simulink model "pndo_org"  (Simulink 10.0)
settings: Solver=ode23tb  StartTime=0.0  StopTime=12  RelTol=1e-3  EnableMultiTasking=on
undefined symbols (not defined in the file): Ts_Control
libraries: powerlib x6, re_lib x1
settings Model: Creator=Student  LastModifiedBy=annonymous
settings DataIOCC: LimitDataPoints=on  SignalLoggingSaveFormat=ModelDataLogs
settings OptimizationCC: ExpressionDepthLimit=2147483647
settings DebuggingCC: SolverPrmCheckMsg=warning  FcnCallInpInsideContextMsg=warning  StateNameClashWarn=warning
settings GRTTargetCC: GeneratePreprocessorConditionals=Disable all
settings ConfigComp: CovExternalEMLEnable=off
settings SimscapeCC: SimscapeNormalizeSystem=off

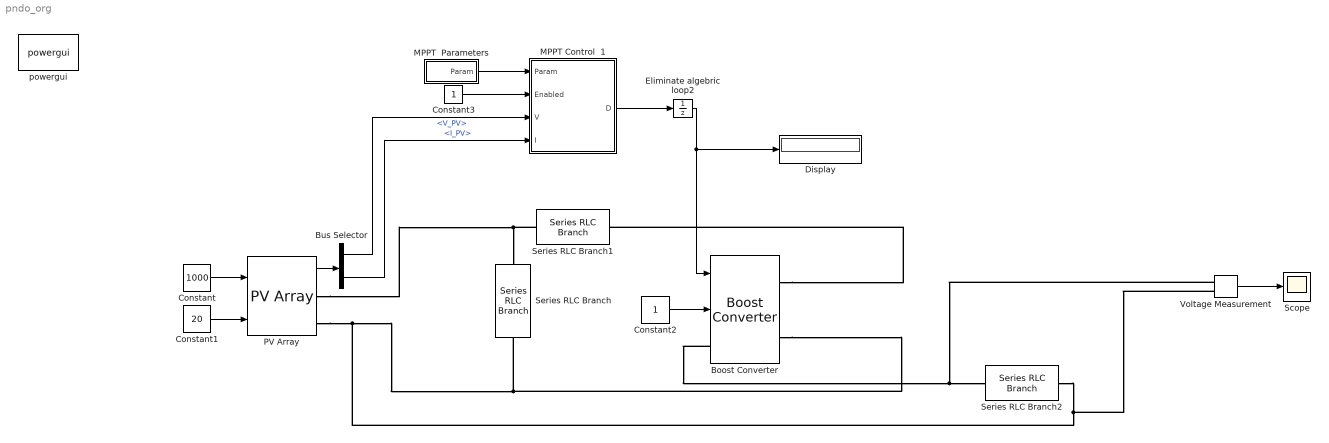
== system pndo_org ==
  Boost Converter : powerlib/Power Electronics/Boost Converter  ModelType=Average model (D-controlled)  Ron=1e-3  Rs=1e6  Cs=inf  Vforward=[0,0]  Ron_Diode=1e-3  Rs_Diode=1e6  Cs_Diode=inf  Vf_Diode=1e-3  Rs_CurrentSource=inf
      settings: SourceProductName=Simscape Electrical  SourceProductBaseCode=PS
  Bus Selector : BusSelector  OutputSignals=V_PV,I_PV
  Constant : Constant  Value=1000
  Constant1 : Constant  Value=20
  Constant2 : Constant
  Constant3 : Constant
  Display : Display
  Eliminate algebric loop2 : UnitDelay  InitialCondition=0.475  SampleTime=Ts_Control  HasFrameUpgradeWarning=on
  MPPT  Parameters : Subsystem
  MPPT Control  1 : MATLAB Function  TreatAsAtomicUnit=on
  PV Array : re_lib/Solar/PV Array  Npar=1  Nser=1  PlotType=array @ 1000 W/m2 & specified temperatures  S_vec="[ 1000  500  100 ]"  Temp_C_vec=[ 45 25 ]  ModuleName=1Soltech 1STH-230-P  PlotWhenSelected=off  Pm=228.735  Ncell=60  Voc=37.1  Isc=8.18  Vm=29.9  Im=7.65  beta_Voc_pc=-0.361  alpha_Isc_pc=0.102  beta_Voc=-0.13393  alpha_Isc=0.008344  IL=8.1897  I0=3.0478e-10  nI=1.0028  Rsh=294.1335  Rs=0.34833  BAL=off  Tc=1e-6  Tfilter=5e-5
      settings: SourceProductName=Simscape Electrical
  Scope : Scope
  Series RLC Branch : powerlib/Elements/Series RLC Branch  LConnTagsString=__new0  RConnTagsString=__new0  BranchType=C  Resistance=1  Inductance=1e-3  SetiL0=off  InitialCurrent=0  Capacitance=100e-6  Setx0=off  InitialVoltage=260  Measurements=None
      settings: SourceProductName=Simscape Electrical
  Series RLC Branch1 : powerlib/Elements/Series RLC Branch  LConnTagsString=__new0  RConnTagsString=__new0  BranchType=RL  Resistance=0.005  Inductance=500e-3  SetiL0=off  InitialCurrent=0  Capacitance=1e-6  Setx0=off  InitialVoltage=0  Measurements=None
      settings: SourceProductName=Simscape Electrical
  Series RLC Branch2 : powerlib/Elements/Series RLC Branch  LConnTagsString=__new0  RConnTagsString=__new0  BranchType=R  Resistance=1000  Inductance=5e-3  SetiL0=off  InitialCurrent=0  Capacitance=1e-6  Setx0=off  InitialVoltage=0  Measurements=None
      settings: SourceProductName=Simscape Electrical
  Voltage Measurement : powerlib/Measurements/Voltage Measurement  PhasorSimulation=off  OutputType=Complex  PSBequivalent=0
      settings: SourceProductName=Simscape Electrical
  powergui : powerlib/powergui  Priority=1  SimulationMode=Continuous  SampleTime=50e-6  frequency=60  Iterations=50  frequencyindice=0  Pbase=100e6  ErrMax=1e-4  UnitsV=kV  UnitsW=MW  buscounter=0  FunctionMessages=off  echomessages=off  EnableUseOfTLC=off  CurrentSourceSwitches=off  DisableSnubberDevices=off  DisableRonSwitches=off  DisableVfSwitches=off  DisplayEquations=off  AutomaticDiscreteSolvers=off  SolverType=Tustin/Backward Euler (TBE)  Interpol=off  ExternalGateDelay=off  methode=off  Ts=0  x0status=blocks  SPID=off  SwTol=0  HookPort=off  NonlinearTolerance=1e-4  nMaxIteration=100  ContinueOnMaxIteration=off  RestoreLinks=warning  ResistiveCurrentMeasurement=off  Frange=[0:2:500]  Ylog=off  Xlog=on  ShowGrid=off  save=off  variable=ZData  structure=0  ZoomFFT=off  StartTime=0.0  cycles=1  DisplayStyle=1  fundamental=60  FreqAxis=off  MaxFrequency=1000  frequencyindicesteady=1  RmsSteady=1  display=off
      settings: SourceProductName=Simscape Electrical
  wires:
  Constant/1 -> PV Array/1
  Constant1/1 -> PV Array/2
  Constant2/1 -> Boost Converter/2
  PV Array/1 -> Bus Selector/1
  Bus Selector/1 -> MPPT Control  1/3(V)  "<V_PV>"
  Bus Selector/2 -> MPPT Control  1/4(I)  "<I_PV>"
  Constant3/1 -> MPPT Control  1/2(Enabled)
  MPPT  Parameters/1(Param) -> MPPT Control  1/1(Param)
  Voltage Measurement/1 -> Scope/1
  MPPT Control  1/1(D) -> Eliminate algebric loop2/1
  Eliminate algebric loop2/1 -> Display/1, Boost Converter/1
  connections:
  PV Array/RConn2 -- Voltage Measurement/LConn2 -- Series RLC Branch2/RConn1 -- Series RLC Branch/RConn1 -- Boost Converter/RConn2
  PV Array/RConn1 -- Series RLC Branch/LConn1 -- Series RLC Branch1/LConn1
  Boost Converter/RConn1 -- Series RLC Branch1/RConn1
  Boost Converter/LConn1 -- Voltage Measurement/LConn1 -- Series RLC Branch2/LConn1

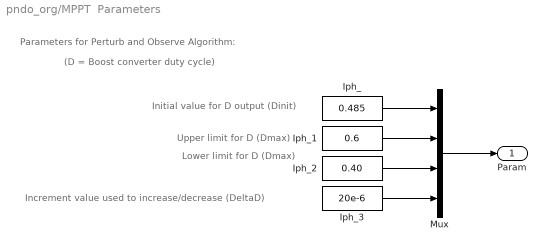
== system pndo_org/MPPT  Parameters ==
  note: Upper limit for D (Dmax)
  note: Increment value used to increase/decrease (DeltaD)
  note: Initial value for D output (Dinit)
  note: (D = Boost converter duty cycle)
  note: Lower limit for D (Dmax)
  note: Parameters for Perturb and Observe Algorithm:
  Iph_ : Constant  Value=0.485
  Iph_1 : Constant  Value=0.6
  Iph_2 : Constant  Value=0.40
  Iph_3 : Constant  Value=20e-6
  Mux : Mux
  Param : Outport
  wires:
  Iph_/1 -> Mux/1
  Iph_1/1 -> Mux/2
  Iph_2/1 -> Mux/3
  Iph_3/1 -> Mux/4
  Mux/1 -> Param/1

== matlab function MPPT Control  1 ==
  settings: updateMethod=DISCRETE  sampleTime=Ts_Control
  data: Param input double; Enabled input double; V input double =V; I input double; D output double
function D  = PandO(Param, Enabled, V, I)
Dinit = Param(1);  
Dmax = Param(2);   
Dmin = Param(3);  
deltaD = Param(4); 
persistent Vold Pold Dold;
dataType = 'double';
if isempty(Vold)
    Vold=0;
    Pold=0;
    Dold=Dinit;
end
P= V*I;
dV= V - Vold;
dP= P - Pold;
if dP ~= 0 & Enabled ~=0
    if dP < 0
        if dV < 0
            D = Dold - deltaD;
        else
            D = Dold + deltaD;
        end
    else
        if dV < 0
            D = Dold + deltaD;
        else
            D = Dold - deltaD;
        end    
    end
else D=Dold;
end
if D >= Dmax | D<= Dmin
    D=Dold;
end
Dold=D;
Vold=V;
Pold=P;
